simulink model "TP4_Trans_PD3"  (R2023b)
settings: Solver=VariableStepAuto  StartTime=0.0  StopTime=0.1  RelTol=1e-3
libraries: spsDiodeLib x6, spsVoltageMeasurementLib x6, spsACVoltageSourceLib x3, spsCurrentMeasurementLib x2, spsGroundLib x1, spsMultimeterLib x1, spsSeriesRLCBranchLib x1, spsThreePhaseTransformerInductanceMatrixTypeTwoWindingsLib x1, spsMeanLib x1, sps_lib x1, dspstat3 x1
settings Model: Creator=HP  LastModifiedBy=HP

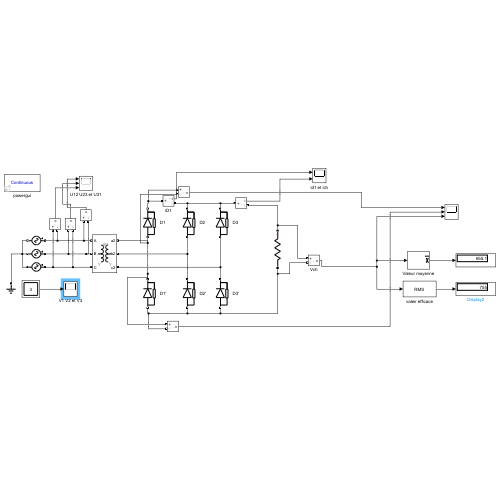
[thumbnail: Simulink's stored preview of the top-level diagram]
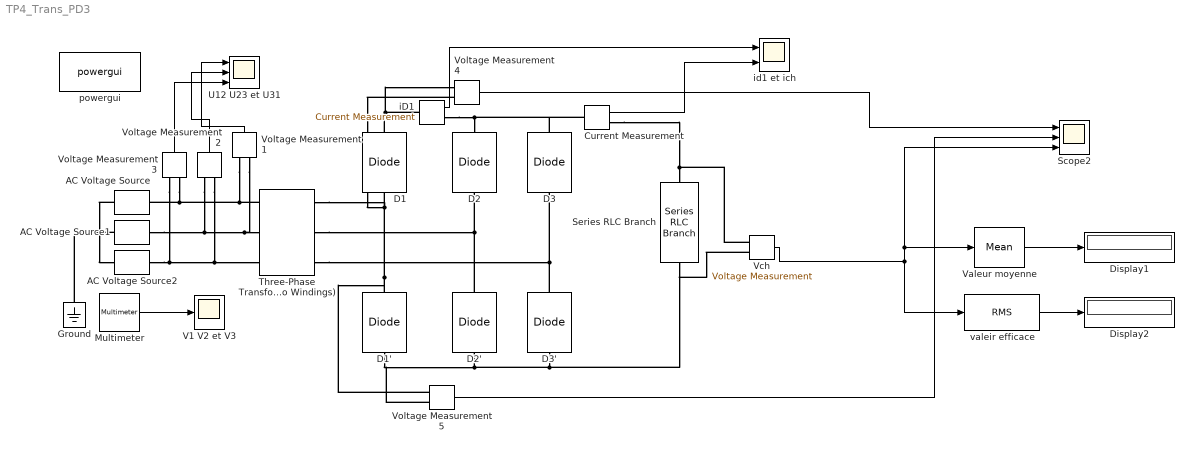
== system TP4_Trans_PD3 ==
  AC Voltage Source : spsACVoltageSourceLib/AC Voltage Source  Amplitude=220  Phase=0  Frequency=50  SampleTime=0  Measurements=Voltage  BusType=swing  Pref=10e3  Qref=0  Qmin=-inf  Qmax=+inf
  AC Voltage Source1 : spsACVoltageSourceLib/AC Voltage Source  Amplitude=220  Phase=120  Frequency=50  SampleTime=0  Measurements=Voltage  BusType=swing  Pref=10e3  Qref=0  Qmin=-inf  Qmax=+inf
  AC Voltage Source2 : spsACVoltageSourceLib/AC Voltage Source  Amplitude=220  Phase=240  Frequency=50  SampleTime=0  Measurements=Voltage  BusType=swing  Pref=10e3  Qref=0  Qmin=-inf  Qmax=+inf
  Current Measurement : spsCurrentMeasurementLib/Current Measurement  PhasorSimulation=off  OutputType=Complex  PSBequivalent=0
  D1 : spsDiodeLib/Diode  Ron=0.001  Lon=0  Vf=0.8  IC=0  UseSnubber=0  Rs=500  Cs=250e-9  Measurements=off
  D1' : spsDiodeLib/Diode  Ron=0.001  Lon=0  Vf=0.8  IC=0  UseSnubber=0  Rs=500  Cs=250e-9  Measurements=off
  D2 : spsDiodeLib/Diode  Ron=0.001  Lon=0  Vf=0.8  IC=0  UseSnubber=0  Rs=500  Cs=250e-9  Measurements=off
  D2' : spsDiodeLib/Diode  Ron=0.001  Lon=0  Vf=0.8  IC=0  UseSnubber=0  Rs=500  Cs=250e-9  Measurements=off
  D3 : spsDiodeLib/Diode  Ron=0.001  Lon=0  Vf=0.8  IC=0  UseSnubber=0  Rs=500  Cs=250e-9  Measurements=off
  D3' : spsDiodeLib/Diode  Ron=0.001  Lon=0  Vf=0.8  IC=0  UseSnubber=0  Rs=500  Cs=250e-9  Measurements=off
  Display1 : Display
  Display2 : Display
  Ground : spsGroundLib/Ground  LConnTagsString=a
  Multimeter : spsMultimeterLib/Multimeter  L=3  sel=[1 2 3]  yselected={}  Gain=[1 1 1]  OutputType=Complex  PlotAtSimulationStop=off  PhasorSimulation=off
  Scope2 : Scope  NumInputPorts=3
  Series RLC Branch : spsSeriesRLCBranchLib/Series RLC Branch  LConnTagsString=__new0  RConnTagsString=__new0  BranchType=R  Resistance=10  Inductance=1e-3  SetiL0=off  InitialCurrent=0  Capacitance=1e-6  Setx0=off  InitialVoltage=0  Measurements=None
  Three-Phase Transformer Inductance Matrix Type (Two Windings) : spsThreePhaseTransformerInductanceMatrixTypeTwoWindingsLib/Three-Phase Transformer Inductance Matrix Type (Two Windings)  CoreType=Three-limb or five-limb core  Winding1Connection=Y  Winding2Connection=Y  AutoTransformer=off  Measurements=None  NominalPower=[100e3, 50]  VLLnom=[200, 400]  WindingResistances=[0.01, 0.01]  NoLoadIexcPos=2  NoLoadPlossPos=1000  ShortCircuitReactancePos=0.06  ShortCircuitReactancePosAuto=0.06  NoLoadIexcZero=100  NoLoadPlossZero=1500  ShortCircuitReactanceZero=0.03  ShortCircuitReactanceZeroAuto=0.03
      settings: LibrarySourceBlock=|
      | sps_lib/Power Grid Elements/Three-Phase Transformer
      | Inductance Matrix Type
      | (Two Windings)
  U12 U23 et U31 : Scope  NumInputPorts=3
  V1 V2 et V3 : Scope
  Valeur moyenne : spsMeanLib/Mean  Freq=60  Vinit=0  Ts=0
  Vch : spsVoltageMeasurementLib/Voltage Measurement  PhasorSimulation=off  OutputType=Complex  PSBequivalent=0
  Voltage Measurement{1..5} (5 alike) : spsVoltageMeasurementLib/Voltage Measurement  PhasorSimulation=off  OutputType=Complex  PSBequivalent=0
  iD1 : spsCurrentMeasurementLib/Current Measurement  PhasorSimulation=off  OutputType=Complex  PSBequivalent=0
  id1 et ich : Scope  NumInputPorts=2
  powergui : sps_lib/powergui  Priority=1  SimulationMode=Continuous  SampleTime=50e-6  frequency=60  Iterations=50  frequencyindice=50  Pbase=100e6  ErrMax=1e-4  UnitsV=kV  UnitsW=MW  buscounter=0  FunctionMessages=off  echomessages=off  EnableUseOfTLC=off  CurrentSourceSwitches=off  DisableSnubberDevices=off  DisableRonSwitches=off  DisableVfSwitches=off  DisplayEquations=off  AutomaticDiscreteSolvers=off  SolverType=Tustin/Backward Euler (TBE)  Interpol=off  ExternalGateDelay=off  methode=off  Ts=100  x0status=blocks  SPID=on  SwTol=0  HookPort=off  NonlinearTolerance=1e-4  nMaxIteration=100  ContinueOnMaxIteration=off  RestoreLinks=warning  ResistiveCurrentMeasurement=off  Frange=[0:2:500]  Ylog=off  Xlog=on  ShowGrid=off  save=off  variable=ZData  structure=0  ZoomFFT=off  StartTime=0.0  cycles=1  DisplayStyle=1  fundamental=60  FreqAxis=off  MaxFrequency=1000  frequencyindicesteady=1  RmsSteady=1  display=off
  valeir efficace : dspstat3/RMS  run=off  directionMode=Each column  dimension=1  InputProcessing=Columns as channels (frame based)  reset_popup=None
  wires:
  valeir efficace/1 -> Display2/1
  Vch/1 -> Valeur moyenne/1, Scope2/3, valeir efficace/1
  Voltage Measurement1/1 -> U12 U23 et U31/1
  Voltage Measurement2/1 -> U12 U23 et U31/2
  Voltage Measurement3/1 -> U12 U23 et U31/3
  Multimeter/1 -> V1 V2 et V3/1
  Voltage Measurement4/1 -> Scope2/1
  Voltage Measurement5/1 -> Scope2/2
  iD1/1 -> id1 et ich/1
  Current Measurement/1 -> id1 et ich/2
  Valeur moyenne/1 -> Display1/1
  connections:
  Vch/LConn1 -- Current Measurement/RConn1 -- Series RLC Branch/LConn1
  D3'/RConn1 -- Three-Phase Transformer Inductance Matrix Type (Two Windings)/RConn3 -- D3/LConn1
  Current Measurement/LConn1 -- D3/RConn1 -- iD1/RConn1 -- D2/RConn1
  D2'/RConn1 -- Three-Phase Transformer Inductance Matrix Type (Two Windings)/RConn2 -- D2/LConn1
  D1'/RConn1 -- Voltage Measurement5/LConn1 -- Voltage Measurement4/LConn2 -- Three-Phase Transformer Inductance Matrix Type (Two Windings)/RConn1 -- D1/LConn1
  D3'/LConn1 -- Vch/LConn2 -- Series RLC Branch/RConn1 -- Voltage Measurement5/LConn2 -- D1'/LConn1 -- D2'/LConn1
  AC Voltage Source/LConn1 -- AC Voltage Source2/LConn1 -- Ground/LConn1 -- AC Voltage Source1/LConn1
  Three-Phase Transformer Inductance Matrix Type (Two Windings)/LConn1 -- Voltage Measurement1/LConn1 -- Voltage Measurement3/LConn2 -- AC Voltage Source/RConn1
  AC Voltage Source1/RConn1 -- Voltage Measurement2/LConn1 -- Voltage Measurement1/LConn2 -- Three-Phase Transformer Inductance Matrix Type (Two Windings)/LConn2
  AC Voltage Source2/RConn1 -- Voltage Measurement3/LConn1 -- Voltage Measurement2/LConn2 -- Three-Phase Transformer Inductance Matrix Type (Two Windings)/LConn3
  D1/RConn1 -- iD1/LConn1 -- Voltage Measurement4/LConn1
